simulink model "gaussianFilter"  (R2024a)
settings: Solver=FixedStepDiscrete  StartTime=0.0  StopTime=1  RelTol=1e-3
libraries: hdlsllib x9, visionsources x1, visionsinks x1, simulink x1
Description:
  | Sobel Edge Detection Using the MATLAB(R) Function Block
  | This example shows how to use HDL Coder(TM) to check,
  | generate, and verify HDL code for a Sobel Edge Detection
  | block built using the MATLAB Function block.
settings Model: FPTRunName=Active  Creator=The MathWorks, Inc.  LastModifiedBy=dskap
settings SolverCC: AlgebraicLoopSolver=TrustRegion
settings DataIOCC: LimitDataPoints=on  SaveFormat=Array  SignalLogging=off  ReturnWorkspaceOutputs=off
settings OptimizationCC: BlockReduction=off  ConditionallyExecuteInputs=off  DefaultParameterBehavior=Inlined  ExpressionDepthLimit=2147483647  InitFltsAndDblsToZero=on  EfficientMapNaN2IntZero=off  LifeSpan=inf
settings DebuggingCC: AlgebraicLoopMsg=error  SaveWithParameterizedLinksMsg=none  UnderspecifiedInitializationDetection=Classic  MergeDetectMultiDrivingBlocksExec=none  SignalResolutionControl=TryResolveAllWithWarning  MultiTaskDSMMsg=warning  MultiTaskCondExecSysMsg=none  SingleTaskRateTransMsg=error  IntegerOverflowMsg=none  ParameterPrecisionLossMsg=none  FcnCallInpInsideContextMsg=warning  UnconnectedInputMsg=warning  UnconnectedOutputMsg=warning  UnconnectedLineMsg=warning  AllowSymbolicDim=off  StateNameClashWarn=warning  StrictBusMsg=ErrorOnBusTreatedAsVector  SFUnexpectedBacktrackingDiag=warning  SFNoUnconditionalDefaultTransitionDiag=warning  SFExecutionAtInitializationDiag=none  IntegerSaturationMsg=none  ArithmeticOperatorsInVariantConditions=warning
settings HardwareCC: ProdBitPerPointer=32  ProdBitPerSizeT=32  ProdBitPerPtrDiffT=32  ProdLargestAtomicFloat=None  ProdIntDivRoundTo=Undefined  ProdEndianess=Unspecified  ProdWordSize=32  ProdHWDeviceType=ASIC/FPGA  TargetHWDeviceType=32-bit Generic  ProdEqTarget=off
settings ModelReferenceCC: EnableRefExpFcnMdlSchedulingChecks=on  PropagateSignalLabelsOutOfModel=off
settings SFSimCC: SimUseLocalCustomCode=off  CustomCodeUndefinedFunction=UseInterfaceOnly
settings RTWCC: RTWUseLocalCustomCode=off  GPUComputeCapability=3.5  DLArmComputeVersion=19.05
settings CodeAppCC: StateflowObjectComments=on
settings GRTTargetCC: TargetFcnLib=ansi_tfl_tmw.mat  TargetLangStandard=C89/C90 (ANSI)  CombineOutputUpdateFcns=off  GRTInterface=on
settings ConfigComp: CovMetricSettings=dw  CovSaveCumulativeToWorkspaceVar=on  CovSaveSingleToWorkspaceVar=on  CovExternalEMLEnable=off

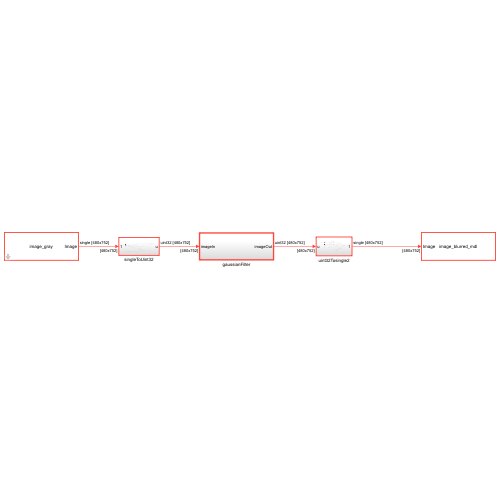
[thumbnail: Simulink's stored preview of the top-level diagram]
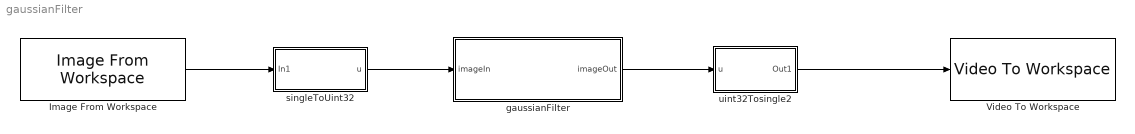
== system gaussianFilter ==
  Image From Workspace : visionsources/Image From Workspace  Tag=vipblks_nd  ImageValue=image_gray  Ts=1  imagePorts=One multidimensional signal  OutPortLabels=R|G|B  ImageDataType=Inherit from 'Value'  Signed=on  WordLength=16  sdImageDataType=sfix(16)  FractionLengthMode=User-defined  FractionLength=15
  Video To Workspace : visionsinks/Video To Workspace  VariableName=image_blurred_mdl  NumInputs=1  DataLimit=1  DecimationFactor=1  LogFi=off  InPortLabels=R|G|B
  gaussianFilter : Subsystem  TreatAsAtomicUnit=on
  singleToUint32 : Subsystem
  uint32Tosingle2 : Subsystem
  wires:
  gaussianFilter/1(imageOut) -> uint32Tosingle2/1(u)
  Image From Workspace/1 -> singleToUint32/1(In1)
  singleToUint32/1(u) -> gaussianFilter/1(imageIn)
  uint32Tosingle2/1(Out1) -> Video To Workspace/1

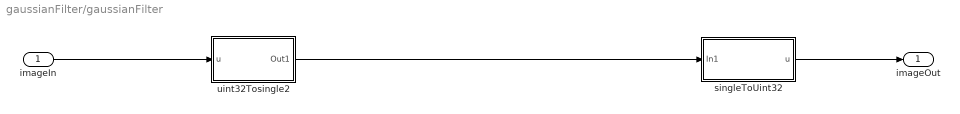
== system gaussianFilter/gaussianFilter ==
  imageIn : Inport
  singleToUint32 : Subsystem
  uint32Tosingle2 : Subsystem
  imageOut : Outport
  wires:
  imageIn/1 -> uint32Tosingle2/1(u)
  uint32Tosingle2/1(Out1) -> singleToUint32/1(In1)
  singleToUint32/1(u) -> imageOut/1

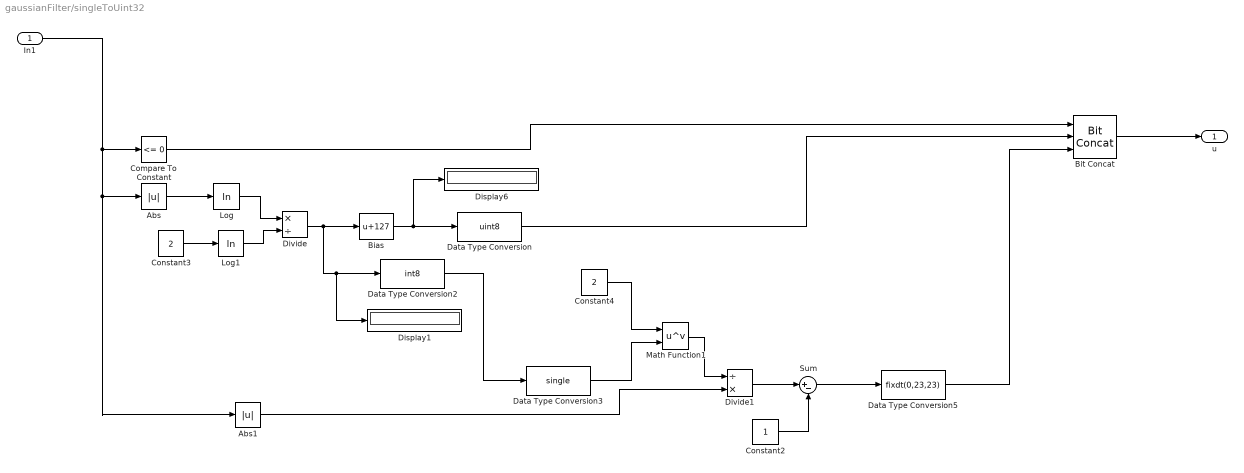
== system gaussianFilter/singleToUint32 ==
  In1 : Inport
  Abs : Abs  SaturateOnIntegerOverflow=off
  Abs1 : Abs  SaturateOnIntegerOverflow=off
  Bias : Bias  Bias=127  SaturateOnIntegerOverflow=off
  Bit Concat : hdlsllib/Logic and Bit Operations/Bit Concat  numInputs=3
  Compare To Constant : simulink/Logic and Bit Operations/Compare To Constant  relop=<=  const=0  OutDataTypeStr=boolean
  Constant2 : Constant  OutDataTypeStr=single  SampleTime=-1
  Constant3 : Constant  Value=2  OutDataTypeStr=single  SampleTime=-1
  Constant4 : Constant  Value=2  OutDataTypeStr=single  SampleTime=-1
  Data Type Conversion : DataTypeConversion  OutDataTypeStr=uint8  SaturateOnIntegerOverflow=off  RndMeth=Floor
  Data Type Conversion2 : DataTypeConversion  OutDataTypeStr=int8  SaturateOnIntegerOverflow=off  RndMeth=Floor
  Data Type Conversion3 : DataTypeConversion  OutDataTypeStr=single  SaturateOnIntegerOverflow=off  RndMeth=Floor
  Data Type Conversion5 : DataTypeConversion  OutDataTypeStr=fixdt(0,23,23)  SaturateOnIntegerOverflow=off  RndMeth=Floor
  Display1 : Display
  Display6 : Display
  Divide : Product  Inputs=*/
  Divide1 : Product  Inputs=/*
  Log : Math  Operator=log
  Log1 : Math  Operator=log
  Math Function1 : Math  Operator=pow
  Sum : Sum  Inputs=|+-
  u : Outport
  wires:
  Divide/1 -> Display1/1, Data Type Conversion2/1, Bias/1
  Bias/1 -> Display6/1, Data Type Conversion/1
  Constant3/1 -> Log1/1
  Abs/1 -> Log/1
  Constant4/1 -> Math Function1/1
  Data Type Conversion3/1 -> Math Function1/2
  Math Function1/1 -> Divide1/1
  Log1/1 -> Divide/2
  Log/1 -> Divide/1
  In1/1 -> Compare To Constant/1, Abs1/1, Abs/1
  Divide1/1 -> Sum/1
  Sum/1 -> Data Type Conversion5/1
  Constant2/1 -> Sum/2
  Abs1/1 -> Divide1/2
  Data Type Conversion2/1 -> Data Type Conversion3/1
  Compare To Constant/1 -> Bit Concat/1
  Data Type Conversion/1 -> Bit Concat/2
  Data Type Conversion5/1 -> Bit Concat/3
  Bit Concat/1 -> u/1

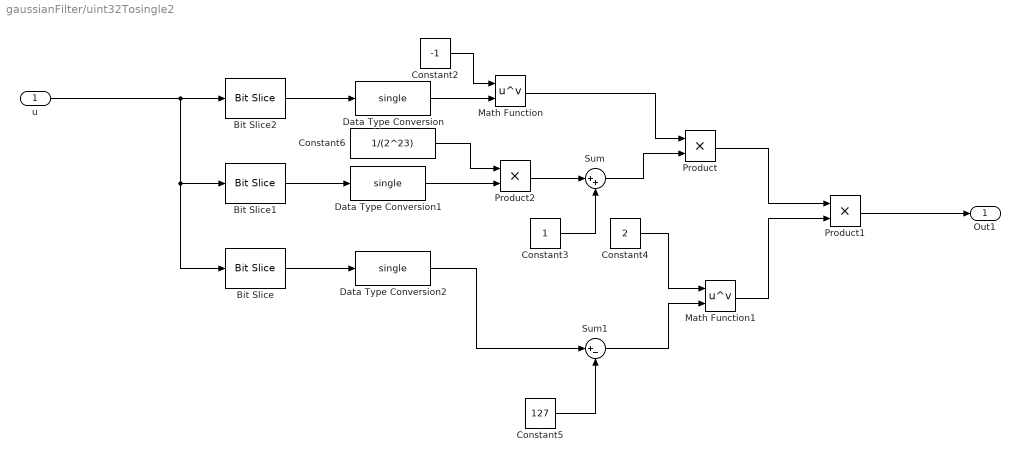
== system gaussianFilter/uint32Tosingle2 ==
  u : Inport
  Bit Slice : hdlsllib/Logic and Bit Operations/Bit Slice  lidx=30  ridx=23
  Bit Slice1 : hdlsllib/Logic and Bit Operations/Bit Slice  lidx=22  ridx=0
  Bit Slice2 : hdlsllib/Logic and Bit Operations/Bit Slice  lidx=31  ridx=31
  Constant2 : Constant  Value=-1  OutDataTypeStr=single  SampleTime=-1
  Constant3 : Constant  OutDataTypeStr=single  SampleTime=-1
  Constant4 : Constant  Value=2  OutDataTypeStr=single  SampleTime=-1
  Constant5 : Constant  Value=127  OutDataTypeStr=single  SampleTime=-1
  Constant6 : Constant  Value=1/(2^23)  OutDataTypeStr=single  SampleTime=-1
  Data Type Conversion : DataTypeConversion  OutDataTypeStr=single  SaturateOnIntegerOverflow=off  RndMeth=Floor
  Data Type Conversion1 : DataTypeConversion  OutDataTypeStr=single  SaturateOnIntegerOverflow=off  RndMeth=Floor
  Data Type Conversion2 : DataTypeConversion  OutDataTypeStr=single  SaturateOnIntegerOverflow=off  RndMeth=Floor
  Math Function : Math  Operator=pow
  Math Function1 : Math  Operator=pow
  Product : Product
  Product1 : Product
  Product2 : Product
  Sum : Sum  Inputs=|++
  Sum1 : Sum  Inputs=|+-
  Out1 : Outport
  wires:
  Product1/1 -> Out1/1
  Bit Slice1/1 -> Data Type Conversion1/1
  Data Type Conversion/1 -> Math Function/2
  Math Function1/1 -> Product1/2
  u/1 -> Bit Slice1/1, Bit Slice/1, Bit Slice2/1
  Constant4/1 -> Math Function1/1
  Product2/1 -> Sum/1
  Bit Slice2/1 -> Data Type Conversion/1
  Sum1/1 -> Math Function1/2
  Constant5/1 -> Sum1/2
  Math Function/1 -> Product/1
  Bit Slice/1 -> Data Type Conversion2/1
  Constant2/1 -> Math Function/1
  Sum/1 -> Product/2
  Product/1 -> Product1/1
  Data Type Conversion1/1 -> Product2/2
  Constant3/1 -> Sum/2
  Data Type Conversion2/1 -> Sum1/1
  Constant6/1 -> Product2/1

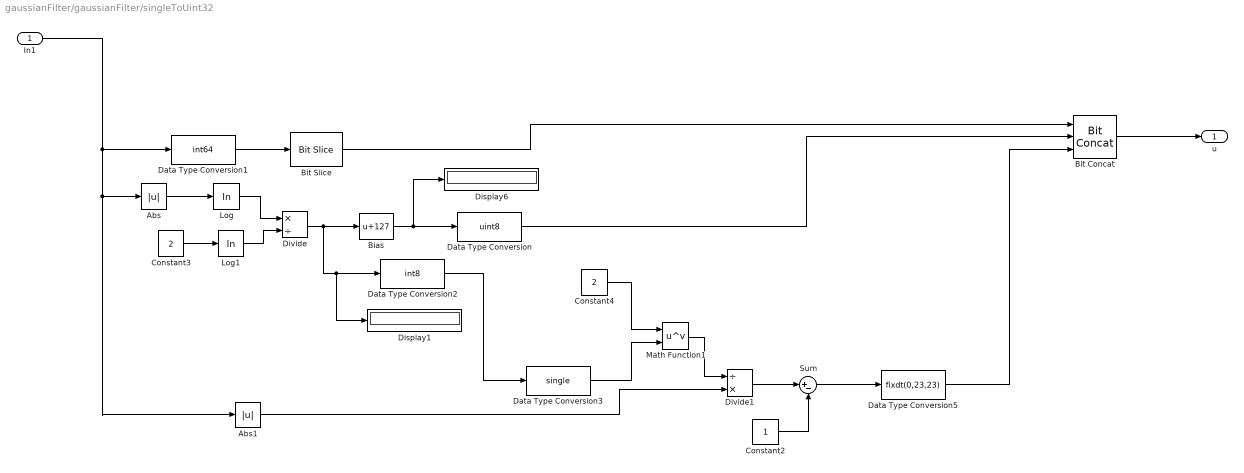
== system gaussianFilter/gaussianFilter/singleToUint32 ==
  In1 : Inport
  Abs : Abs  SaturateOnIntegerOverflow=off
  Abs1 : Abs  SaturateOnIntegerOverflow=off
  Bias : Bias  Bias=127  SaturateOnIntegerOverflow=off
  Bit Concat : hdlsllib/Logic and Bit Operations/Bit Concat  numInputs=3
  Bit Slice : hdlsllib/Logic and Bit Operations/Bit Slice  lidx=63  ridx=63
  Constant2 : Constant  OutDataTypeStr=single  SampleTime=-1
  Constant3 : Constant  Value=2  OutDataTypeStr=single  SampleTime=-1
  Constant4 : Constant  Value=2  OutDataTypeStr=single  SampleTime=-1
  Data Type Conversion : DataTypeConversion  OutDataTypeStr=uint8  SaturateOnIntegerOverflow=off  RndMeth=Floor
  Data Type Conversion1 : DataTypeConversion  OutDataTypeStr=int64  SaturateOnIntegerOverflow=off  RndMeth=Floor
  Data Type Conversion2 : DataTypeConversion  OutDataTypeStr=int8  SaturateOnIntegerOverflow=off  RndMeth=Floor
  Data Type Conversion3 : DataTypeConversion  OutDataTypeStr=single  SaturateOnIntegerOverflow=off  RndMeth=Floor
  Data Type Conversion5 : DataTypeConversion  OutDataTypeStr=fixdt(0,23,23)  SaturateOnIntegerOverflow=off  RndMeth=Floor
  Display1 : Display
  Display6 : Display
  Divide : Product  Inputs=*/
  Divide1 : Product  Inputs=/*
  Log : Math  Operator=log
  Log1 : Math  Operator=log
  Math Function1 : Math  Operator=pow
  Sum : Sum  Inputs=|+-
  u : Outport
  wires:
  Divide/1 -> Display1/1, Data Type Conversion2/1, Bias/1
  Bias/1 -> Display6/1, Data Type Conversion/1
  Constant3/1 -> Log1/1
  Abs/1 -> Log/1
  Constant4/1 -> Math Function1/1
  Data Type Conversion3/1 -> Math Function1/2
  Math Function1/1 -> Divide1/1
  Log1/1 -> Divide/2
  Log/1 -> Divide/1
  In1/1 -> Data Type Conversion1/1, Abs1/1, Abs/1
  Divide1/1 -> Sum/1
  Sum/1 -> Data Type Conversion5/1
  Constant2/1 -> Sum/2
  Abs1/1 -> Divide1/2
  Data Type Conversion2/1 -> Data Type Conversion3/1
  Data Type Conversion1/1 -> Bit Slice/1
  Data Type Conversion/1 -> Bit Concat/2
  Data Type Conversion5/1 -> Bit Concat/3
  Bit Concat/1 -> u/1
  Bit Slice/1 -> Bit Concat/1

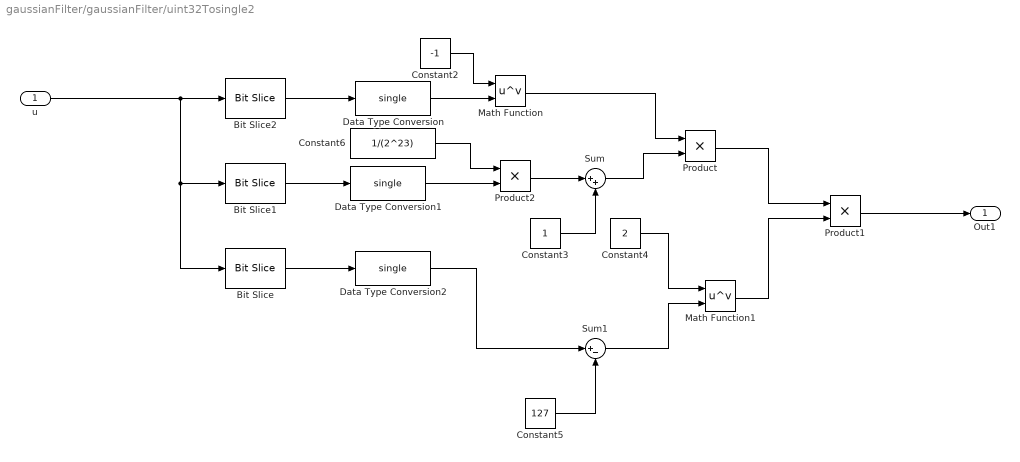
== system gaussianFilter/gaussianFilter/uint32Tosingle2 ==
  u : Inport
  Bit Slice : hdlsllib/Logic and Bit Operations/Bit Slice  lidx=30  ridx=23
  Bit Slice1 : hdlsllib/Logic and Bit Operations/Bit Slice  lidx=22  ridx=0
  Bit Slice2 : hdlsllib/Logic and Bit Operations/Bit Slice  lidx=31  ridx=31
  Constant2 : Constant  Value=-1  OutDataTypeStr=single  SampleTime=-1
  Constant3 : Constant  OutDataTypeStr=single  SampleTime=-1
  Constant4 : Constant  Value=2  OutDataTypeStr=single  SampleTime=-1
  Constant5 : Constant  Value=127  OutDataTypeStr=single  SampleTime=-1
  Constant6 : Constant  Value=1/(2^23)  OutDataTypeStr=single  SampleTime=-1
  Data Type Conversion : DataTypeConversion  OutDataTypeStr=single  SaturateOnIntegerOverflow=off  RndMeth=Floor
  Data Type Conversion1 : DataTypeConversion  OutDataTypeStr=single  SaturateOnIntegerOverflow=off  RndMeth=Floor
  Data Type Conversion2 : DataTypeConversion  OutDataTypeStr=single  SaturateOnIntegerOverflow=off  RndMeth=Floor
  Math Function : Math  Operator=pow
  Math Function1 : Math  Operator=pow
  Product : Product
  Product1 : Product
  Product2 : Product
  Sum : Sum  Inputs=|++
  Sum1 : Sum  Inputs=|+-
  Out1 : Outport
  wires:
  Product1/1 -> Out1/1
  Bit Slice1/1 -> Data Type Conversion1/1
  Data Type Conversion/1 -> Math Function/2
  Math Function1/1 -> Product1/2
  u/1 -> Bit Slice1/1, Bit Slice/1, Bit Slice2/1
  Constant4/1 -> Math Function1/1
  Product2/1 -> Sum/1
  Bit Slice2/1 -> Data Type Conversion/1
  Sum1/1 -> Math Function1/2
  Constant5/1 -> Sum1/2
  Math Function/1 -> Product/1
  Bit Slice/1 -> Data Type Conversion2/1
  Constant2/1 -> Math Function/1
  Sum/1 -> Product/2
  Product/1 -> Product1/1
  Data Type Conversion1/1 -> Product2/2
  Constant3/1 -> Sum/2
  Data Type Conversion2/1 -> Sum1/1
  Constant6/1 -> Product2/1
